simulink model "SG__REF_I"  (R2022b)
settings: Solver=FixedStepAuto  StartTime=0.0  StopTime=Inf  RelTol=1e-3  EnableMultiTasking=on
model workspace (MAT data in the model file):
  N_trig = Simulink.Parameter
  N_trig.Value = 4
  N_trig.Description = 'number of samples for triggered pulse for recording'
  N_trig.DataType = 'auto'
  N_trig.Complexity = 'real'
  N_trig.Dimensions = [1 1]
  a_1 = Simulink.Parameter
  a_1.Value = [1 1 1]
  a_1.DataType = 'auto'
  a_1.Complexity = 'real'
  a_1.Dimensions = [1 3]
  b_1 = Simulink.Parameter
  b_1.Value = [0.5 0.5 0.5]
  b_1.DataType = 'auto'
  b_1.Complexity = 'real'
  b_1.Dimensions = [1 3]
  enable_source = Simulink.Parameter
  enable_source.Value = 0
  enable_source.DataType = 'boolean'
  enable_source.Complexity = 'real'
  enable_source.Dimensions = [1 1]
  freq_fin = Simulink.Parameter
  freq_fin.Value = 1200
  freq_fin.DataType = 'auto'
  freq_fin.Complexity = 'real'
  freq_fin.Dimensions = [1 1]
  freq_ini = Simulink.Parameter
  freq_ini.Value = 150
  freq_ini.DataType = 'auto'
  freq_ini.Complexity = 'real'
  freq_ini.Dimensions = [1 1]
  k_1 = Simulink.Parameter
  k_1.Value = [0 0 0]
  k_1.DataType = 'auto'
  k_1.Complexity = 'real'
  k_1.Dimensions = [1 3]
  rec = Simulink.Parameter
  rec.Value = 0
  rec.DataType = 'boolean'
  rec.Complexity = 'real'
  rec.Dimensions = [1 1]
  src_select = Simulink.Parameter
  src_select.Value = 0
  src_select.DataType = 'auto'
  src_select.Complexity = 'real'
  src_select.Dimensions = [1 1]
  sweep_gain = Simulink.Parameter
  sweep_gain.Value = 0.02
  sweep_gain.DataType = 'auto'
  sweep_gain.Complexity = 'real'
  sweep_gain.Dimensions = [1 1]
  tmax = Simulink.Parameter
  tmax.Value = 10
  tmax.DataType = 'auto'
  tmax.Complexity = 'real'
  tmax.Dimensions = [1 1]
  ts_rec = Simulink.Parameter
  ts_rec.Value = 0.0001
  ts_rec.DataType = 'auto'
  ts_rec.Complexity = 'real'
  ts_rec.Dimensions = [1 1]
undefined symbols (not defined in the file): Ended, Single
libraries: simulink x3, speedgoatlib_IO135 x2, hdlsllib x2, speedgoatlib_IO104 x2, slrealtimeloglib x1, dspsigops x1, slrealtimetgmanagement x1
settings Model: SimulationMode=external  DataflowThreadingImplementation=Pthreads  Creator=padlewsk  LastModifiedBy=padlewsk
settings SolverCC: ConcurrentTasks=on  AlgebraicLoopSolver=TrustRegion  PositivePriorityOrder=on  AutoInsertRateTranBlk=on
settings DataIOCC: SaveFormat=StructureWithTime
settings OptimizationCC: GainParamInheritBuiltInType=on  RollThreshold=9  EfficientFloat2IntCast=on  SimCompilerOptimization=on
settings DebuggingCC: TasksWithSamePriorityMsg=none  UnconnectedInputMsg=warning  UnconnectedOutputMsg=warning  UnconnectedLineMsg=warning
settings HardwareCC: ProdBitPerLong=64  ProdLongLongMode=on  ProdHWDeviceType=Intel->x86-64 (Linux 64)
settings ModelReferenceCC: EnableRefExpFcnMdlSchedulingChecks=on  ModelReferenceNumInstancesAllowed=Single
settings RTWCC: Description=Simulink Real-Time  SystemTargetFile=slrealtime.tlc  TemplateMakefile=slrealtime_default_tmf  Toolchain=Simulink Real-Time Toolchain  BuildConfiguration=Faster Runs  CodeExecutionProfiling=on  TargetLang=C++

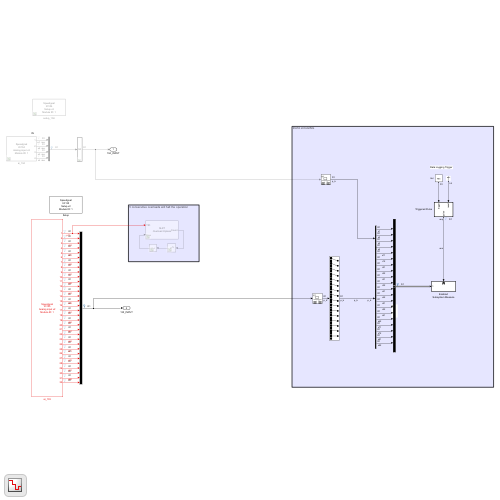
[thumbnail: Simulink's stored preview of the top-level diagram]
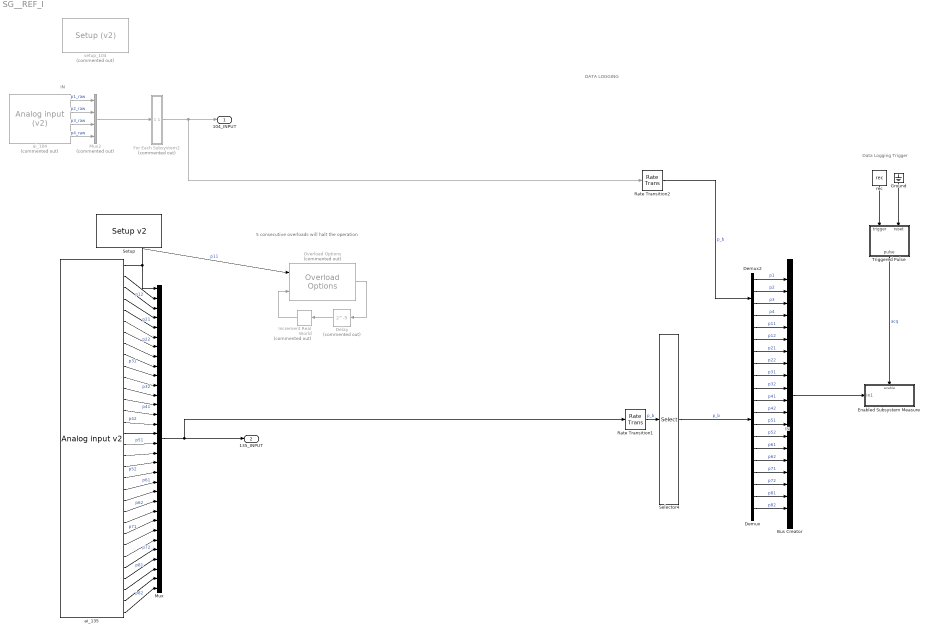
== system SG__REF_I ==
  note: DATA LOGGING
  note: IN
  note: 5 consecutive overloads will halt the operation
  note: Data Logging Trigger
  note: IN
  Bus Creator : BusCreator  Inputs=20
  Delay : Delay  Commented=on  DelayLength=5
  Demux : Demux  Outputs=16
  Demux2 : Demux
  Enabled Subsystem Measure : Subsystem
  For Each Subsystem2 : Subsystem  Commented=on  TreatAsAtomicUnit=on
  Ground : Ground
  Increment Real World : simulink/Additional Math & Discrete/Additional Math: Increment - Decrement/Increment Real World  Commented=on
  Mux : Mux  Inputs=32
  Mux2 : Mux  Commented=on
  Overload Options : slrealtimetgmanagement/Overload Options  Commented=on  startupDur=1  startupDurSrc=Tunable Parameter  maxOverload=0  maxOverloadSrc=Input Port  TETFlag=off
  Rate Transition1 : RateTransition
  Rate Transition2 : RateTransition
  Selector4 : Selector  InputPortWidth=32  IndexOptions=Index vector (dialog)  Indices=[1:2:32]  OutputSizes=1
  Setup : speedgoatlib_IO135/Setup v2   parPciSlot=-1  parModuleId=1  parInterModuleSync=None  parConvClockBaseRate=60MHz  parConvClock1Divider=20000  parConvClock2Divider=20000  parFrameTriggerEnable=off  parFrameTriggerDivider=10  parConvClock1BaseRate=3  parConvClock2BaseRate=3  parFrameTriggerClock=1  parAdcChannels=[1:32]  parAdcRange1=+-5V  parAdcRange2=+-5V  parAdcRange3=+-5V  parAdcRange4=+-5V  parAdcVoltageRange=[1 1 1 1]  parAdcOversampling1=None  parAdcOversampling2=None  parAdcOversampling3=None  parAdcOversampling4=None  parAdcOversamplRate=[1 1 1 1]  parAdcAutoCorrection=on  parAdcContSampling=off  parAdcDmaEnable=off  parAdcDmaClock=Clock 1  parAdcFrameSize_=100  parAdcSampleTime_=-1  parAdcActiveDmaDevices=[1 1 1 1]  parAdcFrameTriggerEnable=0  parAdcFrameSize=100  parAdcSampleTime=0.0333333333333333  parDacChannels=[1:16]  parDacInitValues=0  parDacReset=1  parDacRange1=+-10V  parDacRange2=+-10V  parDacRange3=+-10V  parDacRange4=+-10V  parDacRange5=+-10V  parDacRange6=+-10V  parDacRange7=+-10V  parDacRange8=+-10V  parDacRange9=+-10V  parDacRange10=+-10V  parDacRange11=+-10V  parDacRange12=+-10V  parDacRange13=+-10V  parDacRange14=+-10V  parDacRange15=+-10V  parDacRange16=+-10V  parDacVoltageRange=[5 5 5 5 5 5 5 5 5 5 5 5 5 5 5 5]  parDacAutoCorrection=on  parDacSyncOut=off  parDacDmaEnable=off  parDacDmaLatency=Until next frame  parDacDmaClock=Clock 1  parDacFrameSize_=100  parDacSampleTime_=-1  parDacActiveDmaDevices=[1 1 1 1]  parDacFrameTriggerEnable=0  parDacFrameSize=100  parDacSampleTime=0.0333333333333333  parDoChannels=[]  parDoInitValues=0  parDoReset=1  parDiChannels=[]  parDiDebounceEnable=off  parDiDebounceTime=0  parDiDebounceValue=0  parDioPullRefFront=Pull-up 3.3V  parDioPullRefRear=Floating
      settings: SourceProductName=Simulink Real-Time: Speedgoat I/O Blockset
  "Triggered Pulse " : Subsystem  TreatAsAtomicUnit=on  mask(Triggered Pulse){N=3000}
      mask prompts: N "Length (N samples)"
      mask help: Generates a single pulse of N samples length
  ai_104 : speedgoatlib_IO104/Analog input (v2)   Commented=on  parModuleId=1  parTs=ts  parPciSlot=-1  parAdChannels=[1,2,3,4]  parAdChannelsSorted=[1,2,3,4]  parAdRange1=+-2.5V  parAdRange2=+-2.5V  parAdCoupling=Single-Ended  parAdFrameSize=1  parAdUseTrigger=off  parAdClockInitiator=Initiator  parAdSampleTime=9.920634921e-07  parTriggerInitiator=Initiator  parTriggerRate=4.161015625e-01
      settings: SourceProductName=Simulink Real-Time: Speedgoat I/O Blockset
  ai_135 : speedgoatlib_IO135/Analog input v2   parModuleId=1  parSampleTime=ts  parPciSlot=-1  parAdcChannels=[1 2 3 4 5 6 7 8 9 10 11 12 13 14 15 16 17 18 19 20 21 22 23 24 25 26 27 28 29 30 31 32]  parAdcVoltageRange=[1 1 1 1]  parAdcOversamplRate=[1 1 1 1]  parAdcContSampling=0  parAdcDmaEnable=0  parAdcActiveDmaDevices=[1 1 1 1]  parAdcFrameSize=100
      settings: SourceProductName=Simulink Real-Time: Speedgoat I/O Blockset
  rec : Constant  Value=rec  SampleTime=-1
  setup_104 : speedgoatlib_IO104/Setup (v2)   Commented=on  parPciSlot=-1  parModuleId=1  parTriggerInitiator=Initiator  parTriggerRate=4.161015625e-01  parCalibrate=off  parAdChannels=[1:4]  parAdRange1=+-2.5V  parAdRange2=+-2.5V  parAdCoupling=Single-Ended  parAdUseTrigger=off  parAdFrameSize=1  parAdClockInitiator=Initiator  parAdSampleTime=9.920634921e-07  parDaSimultaneous=on  parDaChannels=[1:4]  parDaChannelsSorted=[1,2,3,4]  parDaInitValue=[0]  parDaReset=[1]  parDaRange=+-10V  parDaUseTrigger=off  parDaFrameSize=1  parDaClockInitiator=Initiator  parDaSampleTime=9.920634921e-07  parDioByte0Dir=Outputs  parDioByte1Dir=Inputs  parDoChannels=[]  parDoInitValues=[0]  parDoReset=[1]  parDiChannels=[]
      settings: SourceProductName=Simulink Real-Time: Speedgoat I/O Blockset
  104_INPUT : Outport
  135_INPUT : Outport  Port=2
  wires:
  ai_104/3 -> Mux2/3  "p3_raw"
  ai_104/2 -> Mux2/2  "p2_raw"
  Mux2/1 -> For Each Subsystem2/1(In1)
  ai_104/1 -> Mux2/1  "p1_raw"
  ai_104/4 -> Mux2/4  "p4_raw"
  ai_135/1 -> Mux/1, Overload Options/1  "p11"
  ai_135/17 -> Mux/17  "p51"
  Mux/1 -> Rate Transition1/1, 135_INPUT/1
  ai_135/4 -> Mux/4
  Increment Real World/1 -> Overload Options/2
  ai_135/9 -> Mux/9  "p31"
  ai_135/26 -> Mux/26
  ai_135/25 -> Mux/25  "p71"
  Delay/1 -> Increment Real World/1
  ai_135/27 -> Mux/27  "p72"
  ai_135/19 -> Mux/19  "p52"
  ai_135/22 -> Mux/22
  ai_135/3 -> Mux/3  "p12"
  ai_135/31 -> Mux/31  "p82"
  ai_135/5 -> Mux/5  "p21"
  ai_135/16 -> Mux/16
  ai_135/24 -> Mux/24
  ai_135/10 -> Mux/10
  ai_135/32 -> Mux/32
  ai_135/6 -> Mux/6
  ai_135/12 -> Mux/12
  ai_135/15 -> Mux/15  "p42"
  ai_135/20 -> Mux/20
  ai_135/18 -> Mux/18
  ai_135/7 -> Mux/7  "p22"
  ai_135/11 -> Mux/11  "p32"
  ai_135/28 -> Mux/28
  ai_135/21 -> Mux/21  "p61"
  ai_135/8 -> Mux/8
  ai_135/23 -> Mux/23  "p62"
  ai_135/30 -> Mux/30
  ai_135/2 -> Mux/2
  ai_135/13 -> Mux/13  "p41"
  ai_135/29 -> Mux/29  "p81"
  ai_135/14 -> Mux/14
  Bus Creator/1 -> Enabled Subsystem Measure/1(In1)
  Demux2/2 -> Bus Creator/2  "p2"
  Demux/5 -> Bus Creator/9  "p31"
  Demux/12 -> Bus Creator/16  "p62"
  Demux/6 -> Bus Creator/10  "p32"
  Ground/1 -> "Triggered Pulse "/2(reset)
  Demux/10 -> Bus Creator/14  "p52"
  Selector4/1 -> Demux/1  "p_b"
  "Triggered Pulse "/1(pulse) -> Enabled Subsystem Measure/Enable  "acq"
  Demux/3 -> Bus Creator/7  "p21"
  Demux/7 -> Bus Creator/11  "p41"
  rec/1 -> "Triggered Pulse "/1(trigger)
  Demux/11 -> Bus Creator/15  "p61"
  Rate Transition1/1 -> Selector4/1  "p_b"
  Demux/9 -> Bus Creator/13  "p51"
  Demux/1 -> Bus Creator/5  "p11"
  Demux/8 -> Bus Creator/12  "p42"
  Demux2/4 -> Bus Creator/4  "p4"
  Demux/14 -> Bus Creator/18  "p72"
  Demux/15 -> Bus Creator/19  "p81"
  Demux/2 -> Bus Creator/6  "p12"
  Demux2/3 -> Bus Creator/3  "p3"
  Demux/13 -> Bus Creator/17  "p71"
  Demux/16 -> Bus Creator/20  "p82"
  Demux2/1 -> Bus Creator/1  "p1"
  Demux/4 -> Bus Creator/8  "p22"
  For Each Subsystem2/1(Out1) -> Rate Transition2/1, 104_INPUT/1
  Overload Options/1 -> Delay/1
  Rate Transition2/1 -> Demux2/1  "p_b"

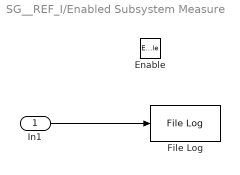
== system SG__REF_I/Enabled Subsystem Measure ==
  In1 : Inport
  Enable : EnablePort
  File Log : slrealtimeloglib/File Log  decimation=1  inputProcessing=Elements as channels (sample based)
  wires:
  In1/1 -> File Log/1

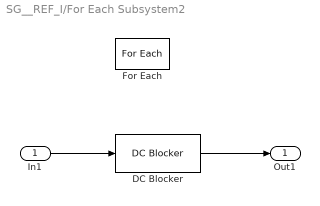
== system SG__REF_I/For Each Subsystem2 ==
  In1 : Inport  Partition=on  PartitionDimension=1  PartitionWidth=1  PartitionOffset=0
  DC Blocker : dspsigops/DC Blocker  Algorithm=FIR  NormalizedBandwidth=0.001  Length=50  Order=6  SimulateUsing=Code generation
      settings: LibrarySourceBlock=dsphdlsupportsigops/DC Blocker
  For Each : ForEach  DisableCoverage=on
  Out1 : Outport  ConcatenationDimension=1
  wires:
  In1/1 -> DC Blocker/1
  DC Blocker/1 -> Out1/1

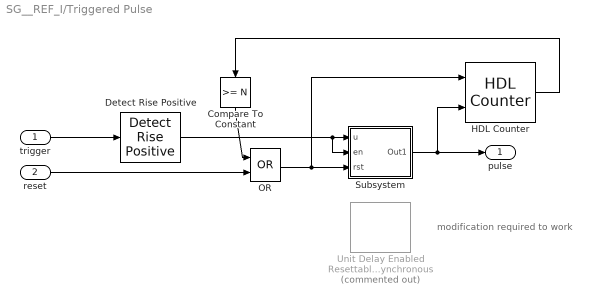
== system SG__REF_I/Triggered Pulse  ==
  note: modification required to work
  trigger : Inport
  reset : Inport  Port=2
  Compare To Constant : simulink/Logic and Bit Operations/Compare To Constant  relop=>=  const=N  OutDataTypeStr=boolean
  Detect Rise Positive : simulink/Logic and Bit Operations/Detect Rise Positive  vinit=0  OutDataTypeStr=boolean
  HDL Counter : hdlsllib/Sources/HDL Counter  CountType=Free running  CountInit=1  CountStep=1  CountMax=25  CountFromType=Initial value  CountFrom=1  CountResetPort=on  CountLoadPort=off  CountEnbPort=on  CountDirPort=off  CountHitOutputPort=off  CountDataType=Unsigned  CountWordLen=32  CountFracLen=0  CountSampTime=1
  OR : Logic  Operator=OR  AllPortsSameDT=off  OutDataTypeStr=boolean
  Subsystem : Subsystem
  Unit Delay Enabled Resettable Synchronous : hdlsllib/Discrete/Unit Delay Enabled Resettable Synchronous  Commented=on  InitialCondition=0.0  SampleTime=-1
  pulse : Outport  VectorParamsAs1DForOutWhenUnconnected=off
  wires:
  OR/1 -> Subsystem/3(rst), HDL Counter/1
  trigger/1 -> Detect Rise Positive/1
  Subsystem/1(Out1) -> HDL Counter/2, pulse/1
  Compare To Constant/1 -> OR/1
  reset/1 -> OR/2
  Detect Rise Positive/1 -> Subsystem/2(en), Subsystem/1(u)
  HDL Counter/1 -> Compare To Constant/1

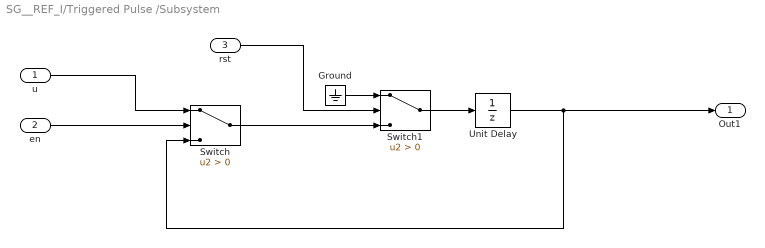
== system SG__REF_I/Triggered Pulse /Subsystem ==
  u : Inport
  en : Inport  Port=2
  rst : Inport  Port=3
  Ground : Ground
  Switch : Switch  Criteria=u2 > Threshold  SaturateOnIntegerOverflow=off  InputSameDT=off
  Switch1 : Switch  Criteria=u2 > Threshold  SaturateOnIntegerOverflow=off  InputSameDT=off
  Unit Delay : UnitDelay  SampleTime=-1  HasFrameUpgradeWarning=on
  Out1 : Outport
  wires:
  Unit Delay/1 -> Switch/3, Out1/1
  en/1 -> Switch/2
  u/1 -> Switch/1
  rst/1 -> Switch1/2
  Ground/1 -> Switch1/1
  Switch1/1 -> Unit Delay/1
  Switch/1 -> Switch1/3
